simulink model "Pacemaker_v6"  (R2025a)
settings: Solver=FixedStepAuto  StartTime=0.0  StopTime=60  FixedStep=1e-3  RelTol=1e-3  EnableMultiTasking=on
undefined symbols (not defined in the file or in its folder): A0, A1, D0, D1, D10, D11, D12, D13, D2, D3, D4, D5, D6, D7, D8, D9, PTA0, PTA1, PTA2, PTB2, PTB23, PTB3, PTB9, PTC16, PTC17, PTC2, PTC3, PTC4, PTD0, PTD1, PTD2, PTD3
libraries: frdmk64flib x22, etargetslib x14, dspstat3 x3
settings Model: ExtModeTrigDuration=5  Creator=emily  LastModifiedBy=tphil
settings SolverCC: AlgebraicLoopSolver=TrustRegion
settings OptimizationCC: EnhancedBackFolding=on  PassReuseOutputArgsAs=Individual arguments  ZeroExternalMemoryAtStartup=off  ZeroInternalMemoryAtStartup=off  MaxStackSize=64  OptimizeBlockOrder=speed  DifferentSizesBufferReuse=on  OptimizationCustomize=off  EfficientTunableParamExpr=on
settings DebuggingCC: ParameterTunabilityLossMsg=error  UnconnectedInputMsg=warning  UnconnectedOutputMsg=warning  UnconnectedLineMsg=warning
settings HardwareCC: ProdBitPerPointer=32.0  ProdBitPerSizeT=32.0  ProdBitPerPtrDiffT=32.0  ProdLargestAtomicInteger=Long  ProdLargestAtomicFloat=Double  ProdWordSize=32.0  ProdHWDeviceType=ARM Compatible->ARM Cortex
settings ModelReferenceCC: EnableRefExpFcnMdlSchedulingChecks=on
settings SFSimCC: MATLABDynamicMemAlloc=off
settings RTWCC: SystemTargetFile=ert.tlc  HardwareBoard=NXP FRDM-K64F  TLCOptions="-aInlineSetEventsForThisBaseRateFcn=TLC_FALSE -aSuppressMultiTaskScheduler=TLC_FALSE  -aRateBasedStepFcn=0"  TemplateMakefile=ert_default_tmf  Toolchain=GNU Tools for ARM Embedded Processors  GPUComputeCapability=3.5  Description=Embedded Coder
settings CodeAppCC: ForceParamTrailComments=on  IgnoreCustomStorageClasses=off  OperatorAnnotations=on  SimulinkDataObjDesc=on  SFDataObjDesc=on  InsertBlockDesc=on
settings ERTTargetCC: ExtModeTransport=0.0  ExtModeStaticAlloc=off  ExtModeMexFile=ext_comm  ExtModeIntrfLevel=Level1  InlinedParameterPlacement=Hierarchical  DynamicArrayContainerType=coder::array

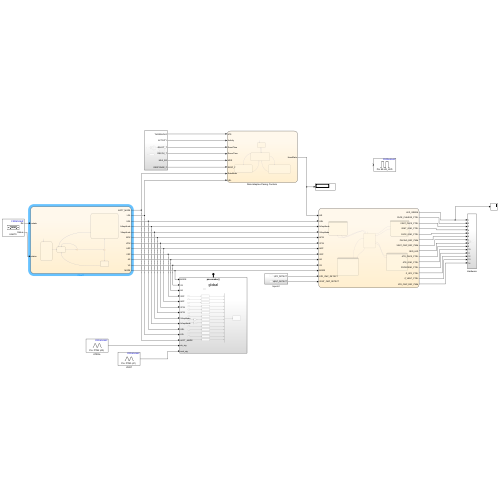
[thumbnail: Simulink's stored preview of the top-level diagram]
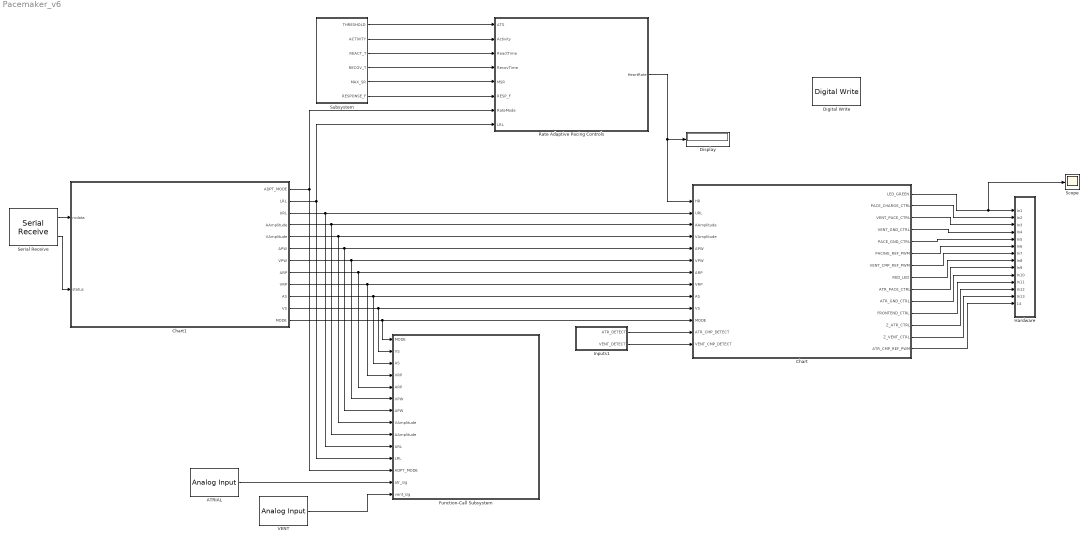
== system Pacemaker_v6 ==
  ATRIAL : frdmk64flib/Analog Input  Whichpin=PTB2 (A0)  SampleTime=-1
  Chart : Stateflow chart  TreatAsAtomicUnit=on
      settings: PortSchema="{\"entries\":[{\"content\":{\"sides\":[{\"content\":{\"connectorIds\":[\"In1\",\"In7\",\"In10\",\"In3\",\"In11\",\"In2\",\"In9\",\"In4\",\"In12\",\"In13\",\"In6\",\"In8\",\"In5\"]},\"type\":\"ConnectorPlacement.EquallySpacedRectSide\",\"uuid\":\"c90d1299-eee1-4468-ae14-5db5d5f4a8fd\"},{\"content\":{\"connectorIds\":[\"Out1\",\"Out2\",\"Out3\",\"Out4\",\"Out5\",\"Out6\",\"Out7\",\"Out8\",\"Out9\",\"Out10\",\"Out11\",\"Out12\",\"Out13\",\"Out14\"],\"side\":\"RIGHT\"},\"type\":\"ConnectorPlacement.EquallySpacedRectSide\",\"uuid\":\"d827a747-ed8c-401d-a91d-ea01b4a5ca13\"},{\"content\":{\"side\":\"TOP\"},\"type\":\"ConnectorPlacement.EquallySpacedRectSide\",\"uuid\":\"7143e8b3-5277-4992-9b61-c0ffb0d94352\"}]},\"type\":\"ConnectorPlacement.EquallySpacedConnector\",\"uuid\":\"d3d4575d-635a-4dca-bcbc-873c423ad5da\"}],\"packageUris\":[\"http://schema.mathworks.com/mf0/Connector/R2020b\"],\"version\":\"1.0\"}"
  Chart1 : Stateflow chart  TreatAsAtomicUnit=on
      settings: PortSchema="{\"entries\":[{\"content\":{\"sides\":[{\"content\":{\"connectorIds\":[\"In1\",\"In2\"]},\"type\":\"ConnectorPlacement.EquallySpacedRectSide\",\"uuid\":\"5fd57579-991f-43e9-bfc1-0ba8facad4d3\"},{\"content\":{\"connectorIds\":[\"Out12\",\"Out1\",\"Out2\",\"Out3\",\"Out4\",\"Out5\",\"Out6\",\"Out7\",\"Out8\",\"Out9\",\"Out10\",\"Out11\"],\"side\":\"RIGHT\"},\"type\":\"ConnectorPlacement.EquallySpacedRectSide\",\"uuid\":\"fb06d67d-cc6b-43c0-93bb-b8d508cd6b5a\"},{\"content\":{\"side\":\"TOP\"},\"type\":\"ConnectorPlacement.EquallySpacedRectSide\",\"uuid\":\"211fcc2e-d126-4388-8a0f-8e8958c4b276\"}]},\"type\":\"ConnectorPlacement.EquallySpacedConnector\",\"uuid\":\"1c3fc2b6-1e97-4470-b124-3e43185d7420\"}],\"packageUris\":[\"http://schema.mathworks.com/mf0/Connector/R2020b\"],\"version\":\"1.0\"}"
  Digital Write : frdmk64flib/Digital Write  Whichpin=BLUE_LED
  Display : Display
  Function-Call Subsystem : Subsystem  TreatAsAtomicUnit=on
  Hardware : Subsystem
  Inputs1 : Subsystem
  "Rate Adaptive Pacing Controls " : Stateflow chart  TreatAsAtomicUnit=on
      settings: PortSchema="{\"entries\":[{\"content\":{\"sides\":[{\"content\":{\"connectorIds\":[\"In1\",\"In2\",\"In3\",\"In4\",\"In7\",\"In8\",\"In5\",\"In6\"]},\"type\":\"ConnectorPlacement.EquallySpacedRectSide\",\"uuid\":\"68d939c0-959f-4d15-809f-f53718f22be8\"},{\"content\":{\"connectorIds\":[\"Out1\"],\"side\":\"RIGHT\"},\"type\":\"ConnectorPlacement.EquallySpacedRectSide\",\"uuid\":\"b191a02a-c2ea-4e78-9182-93b9f8515fb3\"},{\"content\":{\"side\":\"TOP\"},\"type\":\"ConnectorPlacement.EquallySpacedRectSide\",\"uuid\":\"a8053d1b-3bd6-4389-8ac2-60febe55737f\"}]},\"type\":\"ConnectorPlacement.EquallySpacedConnector\",\"uuid\":\"d7a10576-e79c-402c-ae25-f1e5870d93ea\"}],\"packageUris\":[\"http://schema.mathworks.com/mf0/Connector/R2020b\"],\"version\":\"1.0\"}"
  Scope : Scope
      settings: ActiveDisplayYMinimum=-0.0034054463670918356  ActiveDisplayYMaximum=0.29452086491942331  DataLoggingVariableName=ScopeData3
  Serial Receive : frdmk64flib/Serial Receive  SCIModule=0  Baudrate=uint32(9600)  Parity=None  StopBits=1  HardwareFlowControl=None  ByteOrder=LittleEndian  DataType=uint8  DataLength=98  BlockingMode=off  OutputStatus=on  SampleTime=0.1
  Subsystem : Subsystem
  VENT : frdmk64flib/Analog Input  Whichpin=PTB3 (A1)  SampleTime=-1
  wires:
  Chart/2(PACE_CHARGE_CTRL) -> Hardware/2(In2)
  Chart/4(VENT_GND_CTRL) -> Hardware/4(In4)
  Chart/12(Z_ATR_CTRL) -> Hardware/12(In12)
  Chart/7(VENT_CMP_REF_PWM) -> Hardware/7(In7)
  Chart/3(VENT_PACE_CTRL) -> Hardware/3(In3)
  Chart/6(PACING_REF_PWM) -> Hardware/6(In6)
  Chart/13(Z_VENT_CTRL) -> Hardware/13(In13)
  Chart/9(ATR_PACE_CTRL) -> Hardware/9(In9)
  Chart/11(FRONTEND_CTRL) -> Hardware/11(In11)
  Chart/8(RED_LED) -> Hardware/8(In8)
  Chart/10(ATR_GND_CTRL) -> Hardware/10(In10)
  Chart/5(PACE_GND_CTRL) -> Hardware/5(In5)
  Chart/1(LED_GREEN) -> Scope/1, Hardware/1(In1)
  Chart/14(ATR_CMP_REF_PWM) -> Hardware/14(14)
  Serial Receive/1 -> Chart1/1(rxdata)
  ATRIAL/1 -> Function-Call Subsystem/13(atr_sig)
  VENT/1 -> Function-Call Subsystem/14(vent_sig)
  Serial Receive/2 -> Chart1/2(status)
  Chart1/12(ADPT_MODE) -> "Rate Adaptive Pacing Controls "/5(RateMode), Function-Call Subsystem/12(ADPT_MODE)
  Chart1/1(LRL) -> "Rate Adaptive Pacing Controls "/6(LRL), Function-Call Subsystem/11(LRL)
  Chart1/2(URL) -> Function-Call Subsystem/10(URL), Chart/7(URL)
  Chart1/3(AAmplitude) -> Function-Call Subsystem/9(AAmplitude), Chart/10(AAmplitude)
  Inputs1/1(ATR_DETECT) -> Chart/8(ATR_CMP_DETECT)
  Inputs1/2(VENT_DETECT) -> Chart/5(VENT_CMP_DETECT)
  Chart1/4(VAmplitude) -> Function-Call Subsystem/8(VAmplitude), Chart/3(VAmplitude)
  Chart1/5(APW) -> Function-Call Subsystem/7(APW), Chart/11(APW)
  Chart1/6(VPW) -> Function-Call Subsystem/6(VPW), Chart/2(VPW)
  Chart1/7(ARP) -> Function-Call Subsystem/5(ARP), Chart/9(ARP)
  Chart1/8(VRP) -> Function-Call Subsystem/4(VRP), Chart/4(VRP)
  Chart1/9(AS) -> Function-Call Subsystem/3(AS), Chart/12(AS)
  Chart1/10(VS) -> Chart/13(VS), Function-Call Subsystem/2(VS)
  Chart1/11(MODE) -> Chart/6(MODE), Function-Call Subsystem/1(MODE)
  Subsystem/5(MAX_SR) -> "Rate Adaptive Pacing Controls "/7(MSR)
  Subsystem/2(ACTIVITY) -> "Rate Adaptive Pacing Controls "/2(Activity)
  Subsystem/1(THRESHOLD) -> "Rate Adaptive Pacing Controls "/1(ATS)
  Subsystem/4(RECOV_T) -> "Rate Adaptive Pacing Controls "/4(RecovTime)
  Subsystem/6(RESPONSE_F) -> "Rate Adaptive Pacing Controls "/8(RESP_F)
  Subsystem/3(REACT_T) -> "Rate Adaptive Pacing Controls "/3(ReactTime)
  "Rate Adaptive Pacing Controls "/1(HeartRate) -> Display/1, Chart/1(HR)

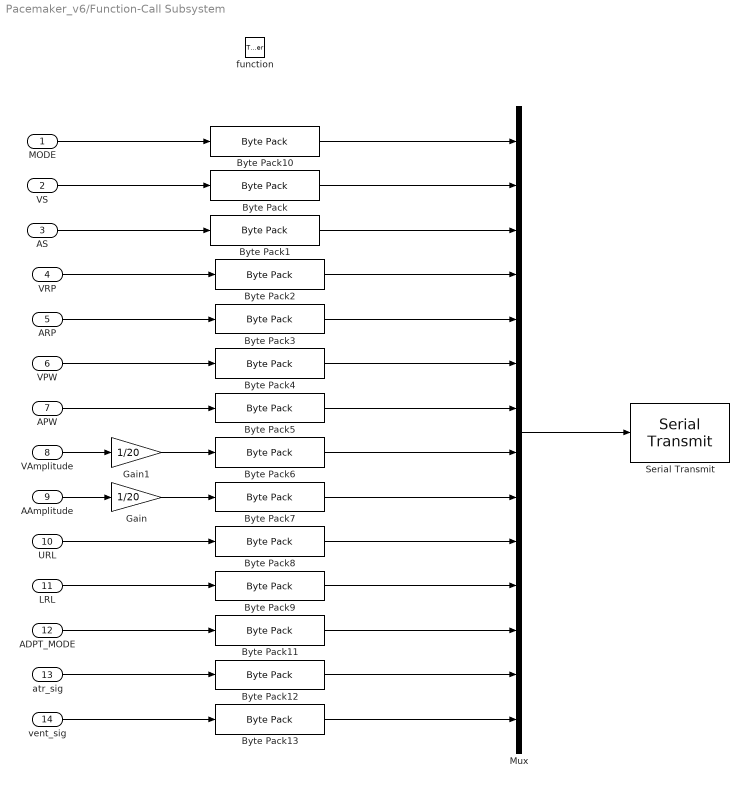
== system Pacemaker_v6/Function-Call Subsystem ==
  MODE : Inport
  VS : Inport  Port=2
  AS : Inport  Port=3
  VRP : Inport  Port=4
  ARP : Inport  Port=5
  VPW : Inport  Port=6
  APW : Inport  Port=7
  VAmplitude : Inport  Port=8
  AAmplitude : Inport  Port=9
  URL : Inport  Port=10
  LRL : Inport  Port=11
  ADPT_MODE : Inport  Port=12
  atr_sig : Inport  Port=13
  vent_sig : Inport  Port=14
  function : TriggerPort  TriggerType=function-call  IsSimulinkFunction=on  FunctionName=pacemaker  VariantControl=(inherit)
  Byte Pack{,1..13} (14 alike) : etargetslib/Byte Pack  datatypes={'double'}  byteAlign=1
  Gain : Gain  Gain=1/20
  Gain1 : Gain  Gain=1/20
  Mux : Mux  Inputs=14
  Serial Transmit : frdmk64flib/Serial Transmit  SCIModule=0  Baudrate=uint32(9600)  Parity=None  StopBits=1  HardwareFlowControl=None  ByteOrder=LittleEndian  BlockingMode=on  OutputStatus=off
  wires:
  VS/1 -> Byte Pack/1
  AS/1 -> Byte Pack1/1
  VRP/1 -> Byte Pack2/1
  Byte Pack/1 -> Mux/2
  Byte Pack1/1 -> Mux/3
  Byte Pack2/1 -> Mux/4
  Byte Pack3/1 -> Mux/5
  Byte Pack4/1 -> Mux/6
  Byte Pack5/1 -> Mux/7
  Byte Pack6/1 -> Mux/8
  Byte Pack7/1 -> Mux/9
  Byte Pack8/1 -> Mux/10
  Byte Pack9/1 -> Mux/11
  ARP/1 -> Byte Pack3/1
  VPW/1 -> Byte Pack4/1
  APW/1 -> Byte Pack5/1
  URL/1 -> Byte Pack8/1
  LRL/1 -> Byte Pack9/1
  Mux/1 -> Serial Transmit/1
  Gain1/1 -> Byte Pack6/1
  VAmplitude/1 -> Gain1/1
  AAmplitude/1 -> Gain/1
  Gain/1 -> Byte Pack7/1
  ADPT_MODE/1 -> Byte Pack11/1
  MODE/1 -> Byte Pack10/1
  Byte Pack10/1 -> Mux/1
  Byte Pack11/1 -> Mux/12
  atr_sig/1 -> Byte Pack12/1
  vent_sig/1 -> Byte Pack13/1
  Byte Pack13/1 -> Mux/14
  Byte Pack12/1 -> Mux/13

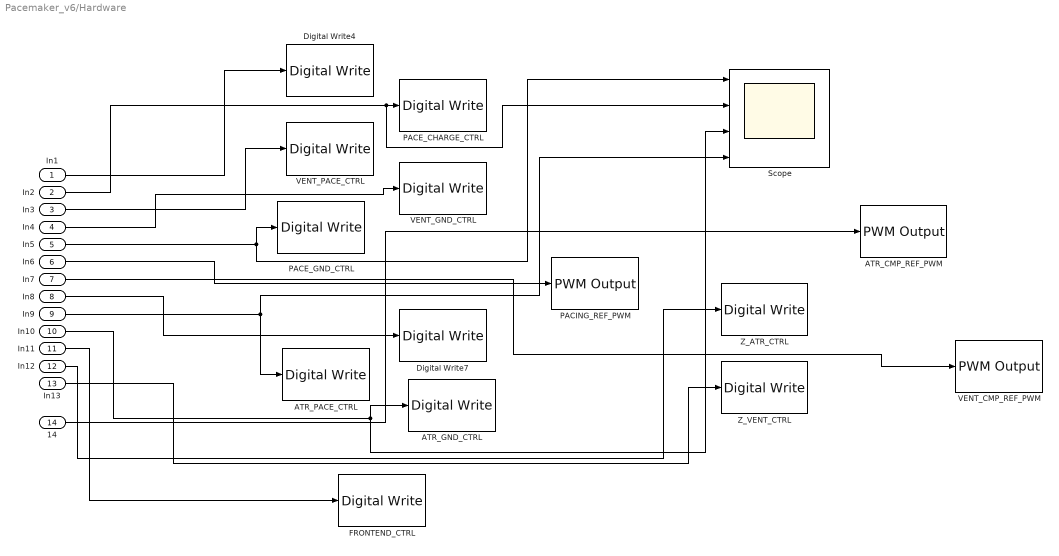
== system Pacemaker_v6/Hardware ==
  In1 : Inport
  In2 : Inport  Port=2
  In3 : Inport  Port=3
  In4 : Inport  Port=4
  In5 : Inport  Port=5
  In6 : Inport  Port=6
  In7 : Inport  Port=7
  In8 : Inport  Port=8
  In9 : Inport  Port=9
  In10 : Inport  Port=10
  In11 : Inport  Port=11
  In12 : Inport  Port=12
  In13 : Inport  Port=13
  14 : Inport  Port=14
  ATR_CMP_REF_PWM : frdmk64flib/PWM Output  Whichpin=PTC2 (D6)  InitialFrequency=2000  InitialDutyCycle=0
  ATR_GND_CTRL : frdmk64flib/Digital Write  Whichpin=PTD2 (D11)
  ATR_PACE_CTRL : frdmk64flib/Digital Write  Whichpin=PTA0 (D8)
  Digital Write4 : frdmk64flib/Digital Write  Whichpin=GREEN_LED
  Digital Write7 : frdmk64flib/Digital Write  Whichpin=RED_LED
  FRONTEND_CTRL : frdmk64flib/Digital Write  Whichpin=PTD1 (D13)
  PACE_CHARGE_CTRL : frdmk64flib/Digital Write  Whichpin=PTB9 (D2)
  PACE_GND_CTRL : frdmk64flib/Digital Write  Whichpin=PTD0 (D10)
  PACING_REF_PWM : frdmk64flib/PWM Output  Whichpin=PTA2 (D5)  InitialFrequency=2000  InitialDutyCycle=30
  Scope : Scope  NumInputPorts=4
      settings: DataLoggingVariableName=ScopeData2
  VENT_CMP_REF_PWM : frdmk64flib/PWM Output  Whichpin=PTA1 (D3)  InitialFrequency=2000  InitialDutyCycle=0
  VENT_GND_CTRL : frdmk64flib/Digital Write  Whichpin=PTD3 (D12)
  VENT_PACE_CTRL : frdmk64flib/Digital Write  Whichpin=PTC4 (D9)
  Z_ATR_CTRL : frdmk64flib/Digital Write  Whichpin=PTB23 (D4)
  Z_VENT_CTRL : frdmk64flib/Digital Write  Whichpin=PTC3 (D7)
  wires:
  In10/1 -> Scope/3, ATR_GND_CTRL/1
  In2/1 -> Scope/2, PACE_CHARGE_CTRL/1
  In6/1 -> PACING_REF_PWM/1
  In4/1 -> VENT_GND_CTRL/1
  In13/1 -> Z_VENT_CTRL/1
  In1/1 -> Digital Write4/1
  In5/1 -> PACE_GND_CTRL/1, Scope/1
  In3/1 -> VENT_PACE_CTRL/1
  In9/1 -> ATR_PACE_CTRL/1, Scope/4
  In8/1 -> Digital Write7/1
  In12/1 -> Z_ATR_CTRL/1
  In11/1 -> FRONTEND_CTRL/1
  14/1 -> ATR_CMP_REF_PWM/1
  In7/1 -> VENT_CMP_REF_PWM/1

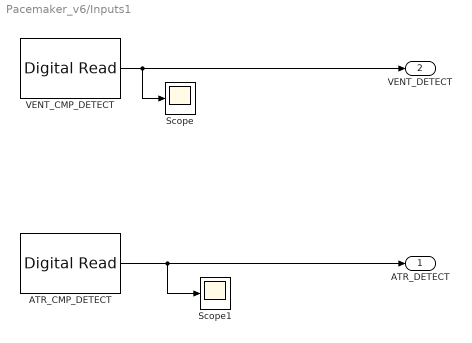
== system Pacemaker_v6/Inputs1 ==
  ATR_CMP_DETECT : frdmk64flib/Digital Read  Whichpin=PTC16 (D0)  SampleTime=-1
  Scope : Scope
      settings: ActiveDisplayYMinimum=0.9  ActiveDisplayYMaximum=1.1
  Scope1 : Scope
      settings: ActiveDisplayYMinimum=0.9  ActiveDisplayYMaximum=1.1
  VENT_CMP_DETECT : frdmk64flib/Digital Read  Whichpin=PTC17 (D1)  SampleTime=inf
  ATR_DETECT : Outport
  VENT_DETECT : Outport  Port=2
  wires:
  VENT_CMP_DETECT/1 -> VENT_DETECT/1, Scope/1
  ATR_CMP_DETECT/1 -> Scope1/1, ATR_DETECT/1

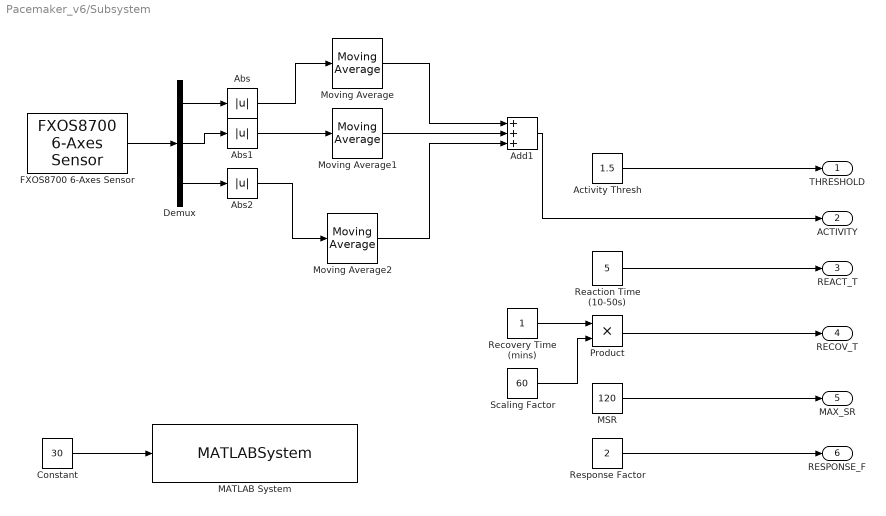
== system Pacemaker_v6/Subsystem ==
  Abs : Abs  SaturateOnIntegerOverflow=off
  Abs1 : Abs  SaturateOnIntegerOverflow=off
  Abs2 : Abs  SaturateOnIntegerOverflow=off
  Activity Thresh : Constant  Value=1.5
  Add1 : Sum  Inputs=+++
  Constant : Constant  Value=30
  Demux : Demux  Outputs=3
  FXOS8700 6-Axes Sensor : frdmk64flib/FXOS8700 6-Axes Sensor  Activesensor=Accelerometer only  ODR=800Hz  HybridODR=400Hz  Accelfullrange=-4g to +4g  SampleTime=-1
  MATLAB System : MATLABSystem  System=ToggleValue  SimulateUsing=Code generation
      mask Type: ToggleValue
  MSR : Constant  Value=120
  Moving Average : dspstat3/Moving Average  Method=Sliding window  ForgettingFactorPort=off  SpecifyWindowLength=on  WindowLength=900  OverlapLength=899  AllowArbitraryInputLength=off  ForgettingFactor=0.9  SimulateUsing=Interpreted execution
  Moving Average1 : dspstat3/Moving Average  Method=Sliding window  ForgettingFactorPort=off  SpecifyWindowLength=on  WindowLength=900  OverlapLength=899  AllowArbitraryInputLength=off  ForgettingFactor=0.9  SimulateUsing=Interpreted execution
  Moving Average2 : dspstat3/Moving Average  Method=Sliding window  ForgettingFactorPort=off  SpecifyWindowLength=on  WindowLength=900  OverlapLength=899  AllowArbitraryInputLength=off  ForgettingFactor=0.9  SimulateUsing=Interpreted execution
  Product : Product
  "Reaction Time (10-50s) " : Constant  Value=5  OutDataTypeStr=double
  Recovery Time (mins) : Constant  OutDataTypeStr=double
  Response Factor : Constant  Value=2  OutDataTypeStr=double
  Scaling Factor : Constant  Value=60
  THRESHOLD : Outport
  ACTIVITY : Outport  Port=2
  REACT_T : Outport  Port=3
  RECOV_T : Outport  Port=4
  MAX_SR : Outport  Port=5
  RESPONSE_F : Outport  Port=6
  wires:
  Moving Average1/1 -> Add1/2
  Scaling Factor/1 -> Product/2
  Demux/3 -> Abs2/1
  FXOS8700 6-Axes Sensor/1 -> Demux/1
  Abs/1 -> Moving Average/1
  Abs2/1 -> Moving Average2/1
  Recovery Time (mins)/1 -> Product/1
  Moving Average/1 -> Add1/1
  Abs1/1 -> Moving Average1/1
  Product/1 -> RECOV_T/1
  Moving Average2/1 -> Add1/3
  Demux/1 -> Abs/1
  Demux/2 -> Abs1/1
  "Reaction Time (10-50s) "/1 -> REACT_T/1
  Activity Thresh/1 -> THRESHOLD/1
  MSR/1 -> MAX_SR/1
  Response Factor/1 -> RESPONSE_F/1
  Constant/1 -> MATLAB System/1
  Add1/1 -> ACTIVITY/1

== stateflow chart Pacemaker_v6/Rate Adaptive Pacing Controls  ==
  state INIT
    entry:
    HeartRate = LRL;
  state RateCheck
    entry:
    sensedRate = LRL + Activity*RESP_F*(MSR-LRL)/2;
  state IncreaseHeartRate
    entry:
    updateBPM = (sensedRate - LRL)/ReactTime/10;
    if (HeartRate <= 120 && HeartRate < sensedRate)
    HeartRate = HeartRate + updateBPM
    end
  state DecreaseHeartRate
    entry:
    updateBPM = (LRL-min(sensedRate, 120))/RecovTime/10;
    if (HeartRate > LRL)
    HeartRate = HeartRate + updateBPM
    end
  (default) -> INIT
  RateCheck -> INIT [order 1] : [RateMode == 0]
  INIT -> RateCheck : [RateMode == 1]
  RateCheck -> IncreaseHeartRate [order 2] : [Activity > ATS]
  RateCheck -> DecreaseHeartRate [order 3] : [(Activity < ATS) || (HeartRate > LRL)]
  IncreaseHeartRate -> RateCheck : after(0.1,sec)
  DecreaseHeartRate -> RateCheck : after(0.1, sec)
  data: ATS input double; Activity input double; ReactTime input double; RecovTime input double; RateMode input double; HeartRate output double; LRL input double; MSR input double; RESP_F input double; sensedRate local; updateBPM local

== stateflow chart Pacemaker_v6/Chart1 ==
  settings: executeAtInitialization=1
  state SET_PARAM
    entry:
    LRL = typecast(rxdata(3:10), 'double');
    URL = typecast(rxdata(11:18), 'double');
    AAmplitude = typecast(rxdata(19:26), 'double')*20;
    APW = typecast(rxdata(27:34), 'double');
    VAmplitude = typecast(rxdata(35:42), 'double')*20;
    VPW = typecast(rxdata(43:50), 'double');
    VRP = typecast(rxdata(51:58), 'double');
    ARP = typecast(rxdata(59:66), 'double');
    AS = typecast(rxdata(67:74), 'double');
    VS = typecast(rxdata(75:82), 'double');
    MODE = typecast(rxdata(83:90), 'double');
    ADPT_MODE = typecast(rxdata(91:98), 'double');
  state INITIAL
    entry:
    LRL = 60;
    URL = 120;
    AAmplitude = 3*20;
    VAmplitude = 3*20;
    ARP = 250;
    VRP = 320;
    APW = 0.4;
    VPW = 0.4;
    AS = 4;
    VS = 3.75;
    MODE = 3;
    ADPT_MODE = 0;
  state STANDBY
    entry:
  state ECHO_PARAM
    entry:
    pacemaker();
  SET_PARAM -> STANDBY
  (junction 21) -> SET_PARAM [order 1] : [rxdata(2) ==hex2dec('55')]
  (default) -> INITIAL
  (junction 20) -> STANDBY [order 2]
  INITIAL -> STANDBY
  STANDBY -> (junction 20) : [status == 0]
  (junction 20) -> (junction 21) [order 1] : [rxdata(1)==hex2dec('16')]
  (junction 21) -> ECHO_PARAM [order 2] : [rxdata(2)==hex2dec('22')]
  ECHO_PARAM -> STANDBY
  data: rxdata input uint8; status input uint8; LRL output double; URL output double; AAmplitude output double; VAmplitude output double; APW output double; VPW output double; ARP output double; VRP output double; AS output double; VS output double; MODE output double; ADPT_MODE output double

== stateflow chart Pacemaker_v6/Chart ==
  state VOO
    entry:
    % Initialize PACE_GND_CTRL and set the PWM amplitude to the Ventricular Amplitude
    PACE_GND_CTRL = 1;
    PACING_REF_PWM = VAmplitude;
    state TIMING
      entry:
      % upon entry into VOO send no pulse
      % and wait for a period - the VPW
      LED_GREEN = 0;
      VENT_PACE_CTRL = 0;
      PACE_CHARGE_CTRL =1;
      VENT_GND_CTRL = 1;
    state PULSE
      entry:
      % upon entry into VOO send no pulse
      % and wait for a period - the VPW
      LED_GREEN = 1;
      PACE_CHARGE_CTRL =0;
      VENT_PACE_CTRL = 1;
      VENT_GND_CTRL = 0;
    (default) -> VOO.TIMING
    VOO.PULSE -> VOO.TIMING : after(VPW, msec)
    VOO.TIMING -> VOO.PULSE : after(60000/(HR) -VPW, msec)
  state AOO
    entry:
    % Initialize PACE_GND_CTRL and set the PWM amplitude to the Atrial Amplitude
    PACE_GND_CTRL = 1;
    PACING_REF_PWM = VAmplitude;
    state TIMING
      entry:
      % upon entry into AOO send no pulse
      % and wait for a period - the APW
      LED_GREEN = 0;
      ATR_PACE_CTRL = 0;
      PACE_CHARGE_CTRL =1;
      ATR_GND_CTRL = 1;
    state PULSE
      entry:
      % after set duration has passed, send
      % a pulse for the APW duration
      LED_GREEN = 1;
      PACE_CHARGE_CTRL =0;
      ATR_GND_CTRL = 0;
      ATR_PACE_CTRL = 1;
    (default) -> AOO.TIMING
    AOO.TIMING -> AOO.PULSE : after(60000/(HR) -APW, msec)
    AOO.PULSE -> AOO.TIMING : after(APW, msec)
  state INITIALIZE
    entry:
    % Initialize inputs
    PACE_CHARGE_CTRL = 0;
    ATR_PACE_CTRL = 0;
    VENT_PACE_CTRL = 0;
    PACE_GND_CTRL = 1;
    ATR_GND_CTRL = 0;
    VENT_GND_CTRL=0;
    FRONTEND_CTRL=1;
    Z_ATR_CTRL = 0;
    Z_VENT_CTRL=0;
  state VVI
    entry:
    % set PACE_GND_CTRL to 1 and the PWM amplitude to Ventricular Amplitude
    PACE_GND_CTRL = 1;
    PACING_REF_PWM = VAmplitude;
    % Set the ATR_CMP_REF_PWM to Ventricular sensitivity
    VENT_CMP_REF_PWM=VS;
    state WAIT
      entry:
      % upon entry wait for signal to be
      % sensed or duration of no pulse
      % to pass
      PACE_CHARGE_CTRL = 1;
      Z_VENT_CTRL=1;
      VENT_PACE_CTRL = 0;
      VENT_GND_CTRL =1;
      %RED_LED = 0;
      %LED_GREEN = 0;
    state PACE
      entry:
      % if no signal was sensed send pulse
      PACE_CHARGE_CTRL = 0;
      Z_VENT_CTRL=0;
      VENT_PACE_CTRL = 1;
      VENT_GND_CTRL = 0;
      %RED_LED = 0;
      %LED_GREEN = 1;
    state REFRACTORY
      entry:
      % if signal was sensed or VPW duration passed
      % wait for VRP duration and go to WAIT state
      PACE_CHARGE_CTRL = 1;
      Z_VENT_CTRL=1;
      VENT_PACE_CTRL = 0;
      VENT_GND_CTRL = 1;
      %RED_LED = 1;
      %LED_GREEN = 0;
    (default) -> VVI.WAIT
    VVI.WAIT -> VVI.PACE [order 1] : after(60000/(HR) -(VPW+VRP), msec)
    VVI.PACE -> VVI.REFRACTORY : after(VPW,msec)
    VVI.WAIT -> VVI.REFRACTORY [order 2] : [VENT_CMP_DETECT==1]
    VVI.REFRACTORY -> VVI.WAIT : after(VRP, msec)
  state AAI
    entry:
    % set PACE_GND_CTRL to 1 and the PWM amplitude to Atrial Amplitude
    PACE_GND_CTRL = 1;
    PACING_REF_PWM = AAmplitude;
    % Set the ATR_CMP_REF_PWM to Atrial sensitivity
    ATR_CMP_REF_PWM=AS;
    state PACE
      entry:
      % if no signal was sensed send pulse
      PACE_CHARGE_CTRL = 0;
      ATR_PACE_CTRL = 1;
      ATR_GND_CTRL = 0;
      RED_LED = 0;
      LED_GREEN = 1;
    state WAIT
      entry:
      % upon entry wait for signal to be
      % sensed or duration of no pulse
      % to pass
      PACE_CHARGE_CTRL = 1;
      ATR_PACE_CTRL = 0;
      ATR_GND_CTRL =1;
      RED_LED = 0;
      LED_GREEN = 0;
    state REFRACTORY
      entry:
      % if signal was sensed or APW duration passed
      % wait for ARP duration and go to WAIT state
      PACE_CHARGE_CTRL = 1;
      ATR_PACE_CTRL = 0;
      ATR_GND_CTRL = 1;
      RED_LED = 1;
      LED_GREEN = 0;
    (default) -> AAI.WAIT
    AAI.WAIT -> AAI.PACE [order 1] : after(60000/(HR) -(APW+ARP), msec)
    AAI.WAIT -> AAI.REFRACTORY [order 2] : [ATR_CMP_DETECT==1]
    AAI.REFRACTORY -> AAI.WAIT : after(ARP, msec)
    AAI.PACE -> AAI.REFRACTORY : after(APW,msec)
  INITIALIZE -> VOO [order 2] : [MODE==2]
  VOO -> INITIALIZE : [MODE~=2]
  AOO -> INITIALIZE : [MODE~=1]
  INITIALIZE -> AOO [order 1] : [MODE==1]
  (default) -> INITIALIZE
  AAI -> INITIALIZE : [MODE~=4]
  INITIALIZE -> VVI [order 4] : [MODE==3]
  VVI -> INITIALIZE : [MODE~=3]
  INITIALIZE -> AAI [order 3] : [MODE==4]
  data: HR input double; VPW input double; LED_GREEN output int16; PACE_CHARGE_CTRL output int16; VENT_PACE_CTRL output int16; VENT_GND_CTRL output int16; PACE_GND_CTRL output int16; PACING_REF_PWM output double; VAmplitude input double; VRP input; VENT_CMP_DETECT input boolean; MODE input double; VENT_CMP_REF_PWM output; RED_LED output; ATR_PACE_CTRL output; ATR_GND_CTRL output; FRONTEND_CTRL output; Z_ATR_CTRL output; Z_VENT_CTRL output; URL input; ATR_CMP_DETECT input; ATR_CMP_REF_PWM output; ARP input; AAmplitude input; APW input; AS input; VS input
